simulink model "twa_parallel"  (Simulink 7.5)
settings: Solver=ode8  StartTime=0.0  StopTime=inf  FixedStep=dt  RelTol=1e-3
PreLoadFcn:
  | addpath('c:\ServoToGo');
  | addpath('d:\Projects\TwistedWireActuator\TWA_parallel_control\init_func')
InitFcn:
  | init_main_twa
  | init_scopes
  | init_twa_homing
  | init_twa_wires
undefined symbols (not defined in the file or in its folder): b_in_w, dt, enc_res, eq_homing, f_in_w, gear_rat, K_d, K_i, K_p, m_in_w, meas_macro_len, N_velocity, p_in_m, rm2w_homing, t_in_w, twa_enc_res, twa_flange_offset, twa_gamma, twa_gear_rat, use_twa, vel_filter_coeffs, velmex_pitch
libraries: xpclib x6, ServoToGo x3, simulink x2, dspswit3 x1
CloseFcn:
  | rtwprivate ssgencode ModelCloseRequest acrochordidae_v1
settings Model: Creator=Roger  LastModifiedBy=ahronoez  BufferReuse=off
settings DataIOCC: LimitDataPoints=off  SaveFormat=StructureWithTime
settings OptimizationCC: BlockReduction=off  OptimizeBlockIOStorage=off  BufferReuse=off  ExpressionFolding=off  LocalBlockOutputs=off  InitFltsAndDblsToZero=on  OptimizeModelRefInitCode=on
settings HardwareCC: ProdIntDivRoundTo=Zero  ProdEndianess=LittleEndian  ProdHWDeviceType=Generic->32-bit x86 compatible
settings RTWCC: SystemTargetFile=xpctargetert.tlc  TemplateMakefile=xpc_ert_tmf  Description=Simulink Real-Time (ERT)  GenerateReport=on  ProcessScript=xpctargetert_make_rtw_hook  IncludeHyperlinkInReport=on  GenerateTraceInfo=on  GenerateTraceReport=on  GenerateTraceReportSl=on  GenerateTraceReportSf=on  GenerateTraceReportEml=on  RTWCompilerOptimization=On
settings xpcTargetERTCC: TargetFcnLib=ansi_tfl_table_tmw.mat  TargetFunctionLibrary=ANSI_C  UtilityFuncGeneration=Auto  ERTMultiwordTypeDef=System defined  ERTCodeCoverageTool=None  ERTMultiwordLength=256  MultiwordLength=2048  GenerateFullHeader=on  GenerateSampleERTMain=off  GenerateTestInterfaces=off  IsPILTarget=off  ModelReferenceCompliant=on  ParMdlRefBuildCompliant=on  CompOptLevelCompliant=on  IncludeMdlTerminateFcn=on  GeneratePreprocessorConditionals=Use local settings  CombineOutputUpdateFcns=off  SuppressErrorStatus=off  ERTFirstTimeCompliant=off  IncludeFileDelimiter=Auto  ERTCustomFileBanners=off  SupportAbsoluteTime=on  LogVarNameModifier=rt_  MatFileLogging=on  MultiInstanceERTCode=off  SupportNonFinite=on  SupportComplex=on  PurelyIntegerCode=off  SupportContinuousTime=on  SupportNonInlinedSFcns=on  SupportVariableSizeSignals=off  EnableShiftOperators=on  ParenthesesLevel=Nominal  PortableWordSizes=off  ModelStepFunctionPrototypeControlCompliant=off  CPPClassGenCompliant=off  AutosarCompliant=off  GenerateASAP2=off  ExtModeTransport=0  ExtModeStaticAlloc=off  ExtModeStaticAllocSize=1000000  ExtModeTesting=off  InlinedParameterPlacement=Hierarchical  TargetOS=BareBoardExample  MultiInstanceErrorCode=Error  RateGroupingCode=on  RootIOFormat=Individual arguments  CoverageDialogOpen=off  ERTFilePackagingFormat=Modular  PreserveExpressionOrder=off  PreserveIfCondition=off  ConvertIfToSwitch=off  PreserveExternInFcnDecls=on  EnableUserReplacementTypes=off  MemSecPackage=--- None ---  MemSecDataConstants=Default  MemSecDataIO=Default  MemSecDataInternal=Default  MemSecDataParameters=Default  MemSecFuncInitTerm=Default  MemSecFuncExecute=Default  GRTInterface=on  GlobalDataDefinition=Auto  GlobalDataReference=Auto  ModuleNamingRule=Unspecified  ERTSrcFileBannerTemplate=ert_code_template.cgt  ERTHdrFileBannerTemplate=ert_code_template.cgt  ERTDataSrcFileTemplate=ert_code_template.cgt  ERTDataHdrFileTemplate=ert_code_template.cgt  ERTCustomFileTemplate=example_file_process.tlc  SignalDisplayLevel=10  ParamTuneLevel=10  InitialValueSource=Model  RTWCAPISignals=off  RTWCAPIParams=on  RTWCAPIStates=off  GenerateErtSFunction=off  RL32ModeModifier=Real-Time  ExtMode=on  ExtModeMexFile=ext_xpc  ExtModeIntrfLevel=Level2 - Open  ExtModeArmWhenConnect=off  RL32LogTETModifier=on  RL32LogBufSizeModifier=100000  RL32IRQSourceModifier=Timer  xPCIRQSourceBoard=None/Other  xPCIOIRQSlot=-1  xpcObjCom=off  xPCGenerateASAP2=off  xPCGenerateXML=off  RL32ObjectName=tg  xPCisDownloadable=off  xPCisDefaultEnv=on  xPCisModelTimeout=on  xPCModelTimeoutSecs=5  xpcDblBuff=off  xPCLoadParamSetFile=off

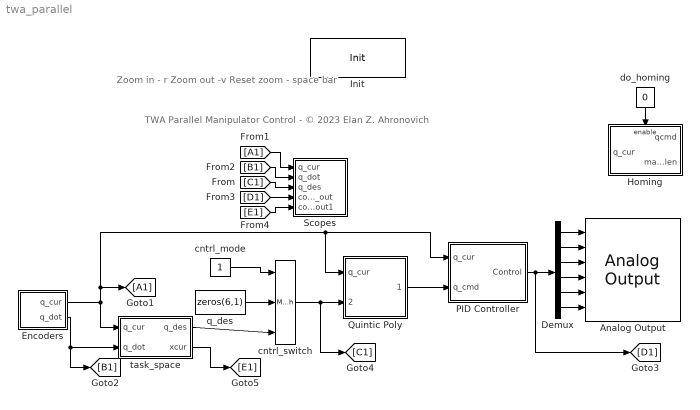
== system twa_parallel ==
  note: TWA Parallel Manipulator Control - © 2023 Elan Z. Ahronovich
  note: Zoom in - r
      | Zoom out -v
      | Reset zoom - space bar
  Analog Output : ServoToGo/Analog Output  Priority=2  channels=[0 1 2 3 4 5]
  Demux : Demux  Outputs=6
  Encoders : Subsystem
  Homing : Subsystem
  Init : ServoToGo/Init  Priority=0  sampletime=dt  baseaddress=0x300  irq_num=5  debug_flag=off  baseaddressD=0
      settings: AttributesFormatString=%<baseaddress>, IRQ: %<irq_num>\n%<sampletime>
  PID Controller : Subsystem
  Quintic Poly : Subsystem
  Scopes : Subsystem
  cntrl_mode : Constant  SampleTime=dt
  cntrl_switch : MultiPortSwitch  Inputs=2  zeroidx=off  OutDataType=fixdt(1, 16)  OutScaling=2^0  SampleTime=dt
  do_homing : Constant  Value=0  SampleTime=dt
  q_des : Constant  Value=zeros(6,1)  SampleTime=dt
  task_space : Subsystem
  wires:
  PID Controller/1(Control) -> Demux/1, [D1]
  Demux/1 -> Analog Output/1
  Demux/2 -> Analog Output/2
  Demux/3 -> Analog Output/3
  Demux/4 -> Analog Output/4
  Demux/5 -> Analog Output/5
  Demux/6 -> Analog Output/6
  Encoders/1(q_cur) -> task_space/1(q_cur), PID Controller/1(q_cur), Quintic Poly/1(q_cur), [A1]
  Encoders/2(q_dot) -> task_space/2(q_dot), [B1]
  q_des/1 -> cntrl_switch/2
  cntrl_mode/1 -> cntrl_switch/1
  Quintic Poly/1(q_cmd) -> PID Controller/2(q_cmd)
  cntrl_switch/1 -> Quintic Poly/2(q_des), [C1]
  do_homing/1 -> Homing/Enable
  task_space/1(q_des) -> cntrl_switch/3
  [C1] -> Scopes/3(q_des)
  [A1] -> Scopes/1(q_cur)
  [B1] -> Scopes/2(q_dot)
  [D1] -> Scopes/4(control_out)
  task_space/2(xcur) -> [E1]
  [E1] -> Scopes/5(control_out1)

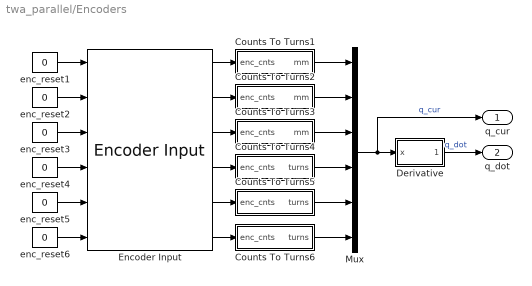
== system twa_parallel/Encoders ==
  Counts To Turns1 : Subsystem
  Counts To Turns2 : Subsystem
  Counts To Turns3 : Subsystem
  Counts To Turns4 : Subsystem
  Counts To Turns5 : Subsystem
  Counts To Turns6 : Subsystem
  Derivative : Subsystem
  Encoder Input : ServoToGo/Encoder Input  Priority=5  channels=[0 1 2 3 4 5 ]  countrev=360
  Mux : Mux  Inputs=6
  enc_reset{1..6} (6 alike) : Constant  Value=0  SampleTime=dt
  q_cur : Outport
  q_dot : Outport  Port=2
  wires:
  Encoder Input/6 -> Counts To Turns6/1(enc_cnts)
  Encoder Input/5 -> Counts To Turns5/1(enc_cnts)
  Encoder Input/4 -> Counts To Turns4/1(enc_cnts)
  Encoder Input/3 -> Counts To Turns3/1(enc_cnts)
  Encoder Input/2 -> Counts To Turns2/1(enc_cnts)
  Mux/1 -> Derivative/1(x), q_cur/1  "q_cur"
  Derivative/1(x_dot) -> q_dot/1  "q_dot"
  Encoder Input/1 -> Counts To Turns1/1(enc_cnts)
  Counts To Turns1/1(mm) -> Mux/1
  enc_reset1/1 -> Encoder Input/1
  Counts To Turns2/1(mm) -> Mux/2
  Counts To Turns3/1(mm) -> Mux/3
  Counts To Turns4/1(turns) -> Mux/4
  Counts To Turns5/1(turns) -> Mux/5
  Counts To Turns6/1(turns) -> Mux/6
  enc_reset2/1 -> Encoder Input/2
  enc_reset3/1 -> Encoder Input/3
  enc_reset4/1 -> Encoder Input/4
  enc_reset5/1 -> Encoder Input/5
  enc_reset6/1 -> Encoder Input/6

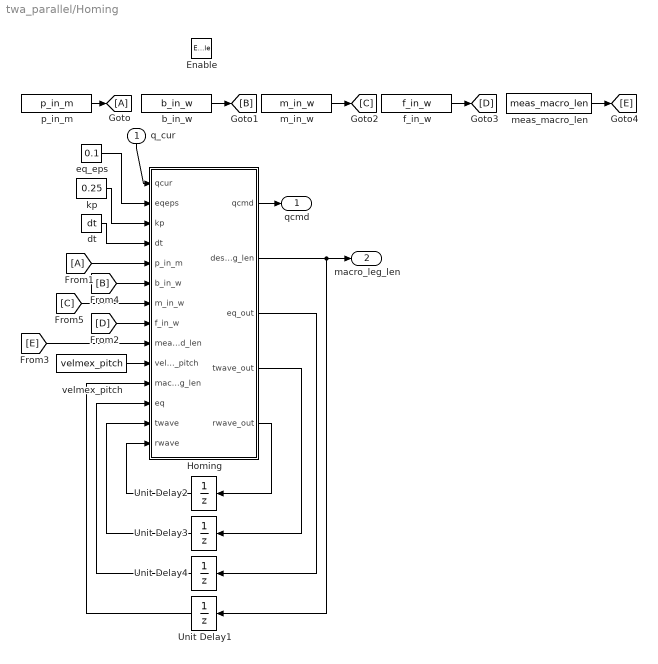
== system twa_parallel/Homing ==
  q_cur : Inport
  Enable : EnablePort
  Homing : Stateflow chart  TreatAsAtomicUnit=on
  Unit Delay1 : UnitDelay  X0=meas_macro_len  SampleTime=dt
  Unit Delay2 : UnitDelay  X0=rm2w_homing  SampleTime=dt
  Unit Delay3 : UnitDelay  X0=zeros(3,1)  SampleTime=dt
  Unit Delay4 : UnitDelay  X0=eq_homing  SampleTime=dt
  b_in_w : Constant  Value=b_in_w  SampleTime=dt
  dt : Constant  Value=dt  SampleTime=dt
  eq_eps : Constant  Value=0.1  SampleTime=dt
  f_in_w : Constant  Value=f_in_w  SampleTime=dt
  kp : Constant  Value=0.25  SampleTime=dt
  m_in_w : Constant  Value=m_in_w  SampleTime=dt
  meas_macro_len : Constant  Value=meas_macro_len  SampleTime=dt
  p_in_m : Constant  Value=p_in_m  SampleTime=dt
  velmex_pitch : Constant  Value=velmex_pitch  SampleTime=dt
  qcmd : Outport
  macro_leg_len : Outport  Port=2
  wires:
  kp/1 -> Homing/3(kp)
  dt/1 -> Homing/4(dt)
  Homing/1(qcmd) -> qcmd/1
  Homing/3(eq_out) -> Unit Delay4/1
  Homing/4(twave_out) -> Unit Delay3/1
  Unit Delay3/1 -> Homing/13(twave)
  Unit Delay4/1 -> Homing/12(eq)
  velmex_pitch/1 -> Homing/10(velmex_pitch)
  Homing/2(des_leg_len) -> Unit Delay1/1, macro_leg_len/1
  Unit Delay1/1 -> Homing/11(macro_leg_len)
  Homing/5(rwave_out) -> Unit Delay2/1
  Unit Delay2/1 -> Homing/14(rwave)
  p_in_m/1 -> [A]
  b_in_w/1 -> [B]
  [A] -> Homing/5(p_in_m)
  [B] -> Homing/6(b_in_w)
  q_cur/1 -> Homing/1(qcur)
  eq_eps/1 -> Homing/2(eqeps)
  [C] -> Homing/7(m_in_w)
  m_in_w/1 -> [C]
  f_in_w/1 -> [D]
  meas_macro_len/1 -> [E]
  [D] -> Homing/8(f_in_w)
  [E] -> Homing/9(measured_len)

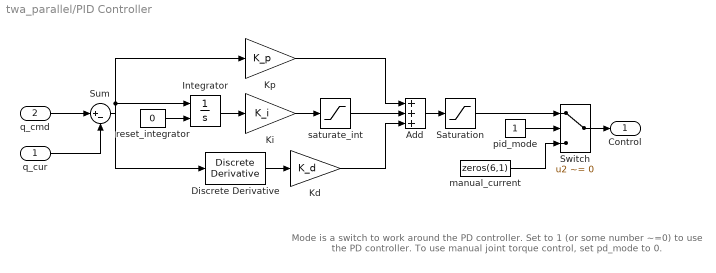
== system twa_parallel/PID Controller ==
  note: Mode is a switch to work around the PD controller.
      | Set to 1 (or some number ~=0) to use the PD
      | controller. To use manual joint torque control, set
      | pd_mode to 0.
  q_cur : Inport
  q_cmd : Inport  Port=2
  Add : Sum  Inputs=+++  SampleTime=dt
  Discrete Derivative : simulink/Discrete/Discrete Derivative  SystemSampleTime=-1  gainval=1.0  ICPrevScaledInput=0.0  OutMin=[]  OutMax=[]  OutDataType=fixdt(1, 16)  OutScaling=2^-10  DoSatur=off
  Integrator : Integrator  ExternalReset=rising
  Kd : Gain  Gain=K_d  SampleTime=dt
  Ki : Gain  Gain=K_i  SampleTime=dt
  Kp : Gain  Gain=K_p  SampleTime=dt
  Saturation : Saturate  UpperLimit=[10,10,10,2,2,2]  LowerLimit=-1*[10,10,10,2,2,2]  LinearizeAsGain=off  SampleTime=dt
  Sum : Sum  Inputs=|+-  SampleTime=dt
  Switch : Switch  Criteria=u2 ~= 0  OutDataType=fixdt(1, 16)  OutScaling=2^0  SampleTime=dt
  manual_current : Constant  Value=zeros(6,1)  SampleTime=dt
  pid_mode : Constant  SampleTime=dt
  reset_integrator : Constant  Value=0  SampleTime=dt
  saturate_int : Saturate  UpperLimit=[5,5,5,.25,0.25,0.25]  LowerLimit=-1*[5,5,5,.25,0.25,0.25]  LinearizeAsGain=off  SampleTime=dt
  Control : Outport
  wires:
  Kp/1 -> Add/1
  Kd/1 -> Add/3
  Add/1 -> Saturation/1
  q_cmd/1 -> Sum/1
  q_cur/1 -> Sum/2
  Switch/1 -> Control/1
  Saturation/1 -> Switch/1
  manual_current/1 -> Switch/3
  Ki/1 -> saturate_int/1
  saturate_int/1 -> Add/2
  Discrete Derivative/1 -> Kd/1
  Integrator/1 -> Ki/1
  Sum/1 -> Kp/1, Discrete Derivative/1, Integrator/1
  pid_mode/1 -> Switch/2
  reset_integrator/1 -> Integrator/2

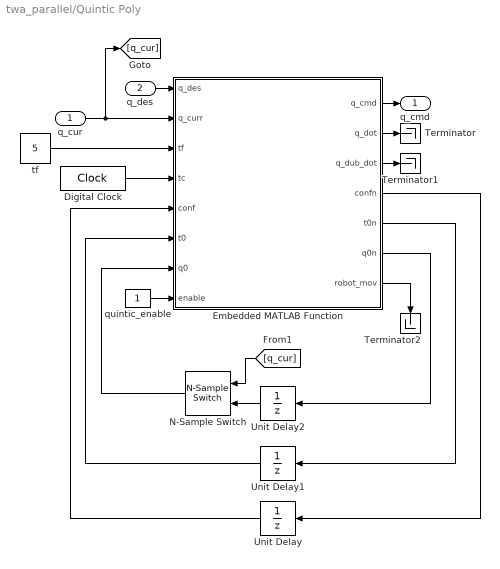
== system twa_parallel/Quintic Poly ==
  q_cur : Inport  OutDataType=fixdt(1, 16)  OutScaling=2^0
  q_des : Inport  Port=2  OutDataType=fixdt(1, 16)  OutScaling=2^0
  Digital Clock : DigitalClock  SampleTime=dt
  Embedded MATLAB Function : Stateflow chart  TreatAsAtomicUnit=on
  N-Sample Switch : dspswit3/N-Sample Switch  SystemSampleTime=-1  N=1  reset=off  TriggerType=Rising edge  Ts=dt
  Terminator : Terminator
  Terminator1 : Terminator
  Terminator2 : Terminator
  Unit Delay : UnitDelay  SampleTime=dt
  Unit Delay1 : UnitDelay  SampleTime=dt
  Unit Delay2 : UnitDelay  X0=zeros(6,1)  SampleTime=dt
  quintic_enable : Constant  SampleTime=dt
  tf : Constant  Value=5  SampleTime=dt
  q_cmd : Outport
  wires:
  Embedded MATLAB Function/4(confn) -> Unit Delay/1
  Unit Delay/1 -> Embedded MATLAB Function/5(conf)
  Embedded MATLAB Function/5(t0n) -> Unit Delay1/1
  Embedded MATLAB Function/6(q0n) -> Unit Delay2/1
  Unit Delay1/1 -> Embedded MATLAB Function/6(t0)
  Digital Clock/1 -> Embedded MATLAB Function/4(tc)
  q_des/1 -> Embedded MATLAB Function/1(q_des)
  tf/1 -> Embedded MATLAB Function/3(tf)
  quintic_enable/1 -> Embedded MATLAB Function/8(enable)
  Embedded MATLAB Function/2(q_dot) -> Terminator/1
  Embedded MATLAB Function/3(q_dub_dot) -> Terminator1/1
  N-Sample Switch/1 -> Embedded MATLAB Function/7(q0)
  Unit Delay2/1 -> N-Sample Switch/2
  [q_cur] -> N-Sample Switch/1
  Embedded MATLAB Function/7(robot_mov) -> Terminator2/1
  Embedded MATLAB Function/1(q_cmd) -> q_cmd/1
  q_cur/1 -> Embedded MATLAB Function/2(q_curr), [q_cur]

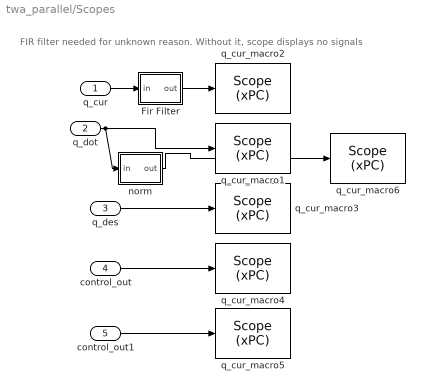
== system twa_parallel/Scopes ==
  note: FIR filter needed for unknown reason.
      |  Without it, scope displays no signals
  q_cur : Inport
  q_dot : Inport  Port=2
  q_des : Inport  Port=3
  control_out : Inport  Port=4
  control_out1 : Inport  Port=5
  Fir Filter : Subsystem
  norm : Subsystem
  q_cur_macro1 : xpclib/Misc./Scope (xPC)   SystemSampleTime=-1  scopeno=2  scopetype=Target  autostart=on  viewmode=Numerical  formatstr=qd_format  grid=on  ylimits=[0,0]  nosamples=25  noprepostsamples=0  interleave=1  triggermode=FreeRun  triggersignal=1  triggerlevel=0.0  triggerslope=Either  triggerscope=1  triggersample=0  filename=data.dat  mode=Lazy  writesize=512  autorestart=off  dynamicfilemode=off  maxwritefilesize=512*1024^2
  q_cur_macro2 : xpclib/Misc./Scope (xPC)   SystemSampleTime=-1  scopeno=1  scopetype=Target  autostart=on  viewmode=Numerical  formatstr=q_format  grid=on  ylimits=[0,0]  nosamples=25  noprepostsamples=0  interleave=1  triggermode=FreeRun  triggersignal=1  triggerlevel=0.0  triggerslope=Either  triggerscope=1  triggersample=0  filename=data.dat  mode=Lazy  writesize=512  autorestart=off  dynamicfilemode=off  maxwritefilesize=512*1024^2
  q_cur_macro3 : xpclib/Misc./Scope (xPC)   SystemSampleTime=-1  scopeno=3  scopetype=Target  autostart=on  viewmode=Numerical  formatstr=qdes_format  grid=on  ylimits=[0,0]  nosamples=25  noprepostsamples=0  interleave=1  triggermode=FreeRun  triggersignal=1  triggerlevel=0.0  triggerslope=Either  triggerscope=1  triggersample=0  filename=data.dat  mode=Lazy  writesize=512  autorestart=off  dynamicfilemode=off  maxwritefilesize=512*1024^2
  q_cur_macro4 : xpclib/Misc./Scope (xPC)   SystemSampleTime=-1  scopeno=4  scopetype=Target  autostart=on  viewmode=Numerical  formatstr=qcmd_format  grid=on  ylimits=[0,0]  nosamples=25  noprepostsamples=0  interleave=1  triggermode=FreeRun  triggersignal=1  triggerlevel=0.0  triggerslope=Either  triggerscope=1  triggersample=0  filename=data.dat  mode=Lazy  writesize=512  autorestart=off  dynamicfilemode=off  maxwritefilesize=512*1024^2
  q_cur_macro5 : xpclib/Misc./Scope (xPC)   SystemSampleTime=-1  scopeno=5  scopetype=Target  autostart=on  viewmode=Numerical  formatstr=xcur_format  grid=on  ylimits=[0,0]  nosamples=25  noprepostsamples=0  interleave=1  triggermode=FreeRun  triggersignal=1  triggerlevel=0.0  triggerslope=Either  triggerscope=1  triggersample=0  filename=data.dat  mode=Lazy  writesize=512  autorestart=off  dynamicfilemode=off  maxwritefilesize=512*1024^2
  q_cur_macro6 : xpclib/Misc./Scope (xPC)   SystemSampleTime=-1  scopeno=6  scopetype=Target  autostart=on  viewmode=Numerical  formatstr='qdot any %8i'  grid=on  ylimits=[0,0]  nosamples=25  noprepostsamples=0  interleave=1  triggermode=FreeRun  triggersignal=1  triggerlevel=0.0  triggerslope=Either  triggerscope=1  triggersample=0  filename=data.dat  mode=Lazy  writesize=512  autorestart=off  dynamicfilemode=off  maxwritefilesize=512*1024^2
  wires:
  Fir Filter/1(out) -> q_cur_macro2/1
  q_cur/1 -> Fir Filter/1(in)
  q_des/1 -> q_cur_macro3/1
  control_out/1 -> q_cur_macro4/1
  control_out1/1 -> q_cur_macro5/1
  q_dot/1 -> norm/1(in), q_cur_macro1/1
  norm/1(out) -> q_cur_macro6/1

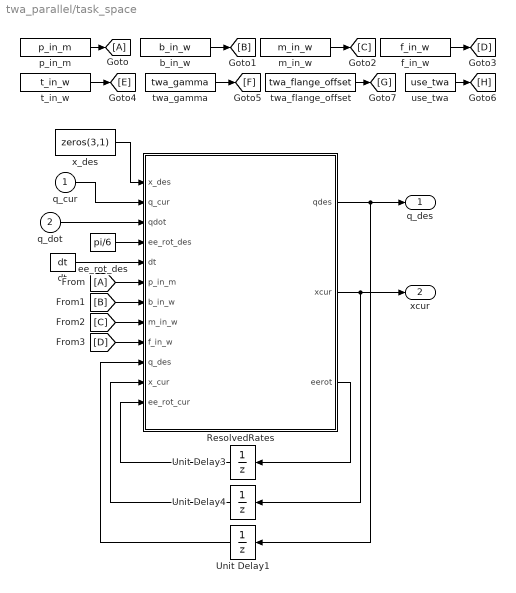
== system twa_parallel/task_space ==
  q_cur : Inport
  q_dot : Inport  Port=2
  ResolvedRates : Stateflow chart  TreatAsAtomicUnit=on
  Unit Delay1 : UnitDelay  X0=zeros(6,1)  SampleTime=dt
  Unit Delay3 : UnitDelay  X0=pi/6  SampleTime=dt
  Unit Delay4 : UnitDelay  X0=zeros(3,1)  SampleTime=dt
  b_in_w : Constant  Value=b_in_w  SampleTime=dt
  dt : Constant  Value=dt  SampleTime=dt
  ee_rot_des : Constant  Value=pi/6  SampleTime=dt
  f_in_w : Constant  Value=f_in_w  SampleTime=dt
  m_in_w : Constant  Value=m_in_w  SampleTime=dt
  p_in_m : Constant  Value=p_in_m  SampleTime=dt
  t_in_w : Constant  Value=t_in_w  SampleTime=dt
  twa_flange_offset : Constant  Value=twa_flange_offset  SampleTime=dt
  twa_gamma : Constant  Value=twa_gamma  SampleTime=dt
  use_twa : Constant  Value=use_twa  SampleTime=dt
  x_des : Constant  Value=zeros(3,1)  SampleTime=dt
  q_des : Outport
  xcur : Outport  Port=2
  wires:
  p_in_m/1 -> [A]
  b_in_w/1 -> [B]
  m_in_w/1 -> [C]
  f_in_w/1 -> [D]
  t_in_w/1 -> [E]
  twa_gamma/1 -> [F]
  twa_flange_offset/1 -> [G]
  use_twa/1 -> [H]
  ResolvedRates/3(eerot) -> Unit Delay3/1
  Unit Delay3/1 -> ResolvedRates/12(ee_rot_cur)
  ResolvedRates/2(xcur) -> Unit Delay4/1, xcur/1
  Unit Delay4/1 -> ResolvedRates/11(x_cur)
  x_des/1 -> ResolvedRates/1(x_des)
  ee_rot_des/1 -> ResolvedRates/4(ee_rot_des)
  [A] -> ResolvedRates/6(p_in_m)
  [B] -> ResolvedRates/7(b_in_w)
  [C] -> ResolvedRates/8(m_in_w)
  [D] -> ResolvedRates/9(f_in_w)
  dt/1 -> ResolvedRates/5(dt)
  ResolvedRates/1(qdes) -> Unit Delay1/1, q_des/1
  q_dot/1 -> ResolvedRates/3(qdot)
  Unit Delay1/1 -> ResolvedRates/10(q_des)
  q_cur/1 -> ResolvedRates/2(q_cur)

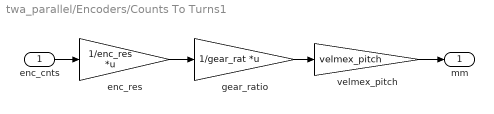
== system twa_parallel/Encoders/Counts To Turns1 ==
  enc_cnts : Inport
  enc_res : Gain  Gain=1/enc_res  Multiplication=Matrix(K*u)  SampleTime=dt
  gear_ratio : Gain  Gain=1/gear_rat  Multiplication=Matrix(K*u)  SampleTime=dt
  velmex_pitch : Gain  Gain=velmex_pitch  SampleTime=dt
  mm : Outport
  wires:
  enc_res/1 -> gear_ratio/1
  enc_cnts/1 -> enc_res/1
  gear_ratio/1 -> velmex_pitch/1
  velmex_pitch/1 -> mm/1

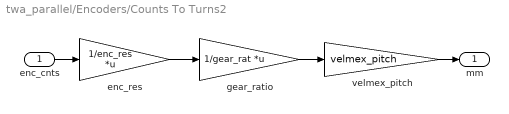
== system twa_parallel/Encoders/Counts To Turns2 ==
  enc_cnts : Inport
  enc_res : Gain  Gain=1/enc_res  Multiplication=Matrix(K*u)  SampleTime=dt
  gear_ratio : Gain  Gain=1/gear_rat  Multiplication=Matrix(K*u)  SampleTime=dt
  velmex_pitch : Gain  Gain=velmex_pitch  SampleTime=dt
  mm : Outport
  wires:
  gear_ratio/1 -> velmex_pitch/1
  enc_cnts/1 -> enc_res/1
  enc_res/1 -> gear_ratio/1
  velmex_pitch/1 -> mm/1

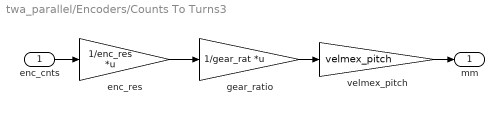
== system twa_parallel/Encoders/Counts To Turns3 ==
  enc_cnts : Inport
  enc_res : Gain  Gain=1/enc_res  Multiplication=Matrix(K*u)  SampleTime=dt
  gear_ratio : Gain  Gain=1/gear_rat  Multiplication=Matrix(K*u)  SampleTime=dt
  velmex_pitch : Gain  Gain=velmex_pitch  SampleTime=dt
  mm : Outport
  wires:
  enc_res/1 -> gear_ratio/1
  enc_cnts/1 -> enc_res/1
  gear_ratio/1 -> velmex_pitch/1
  velmex_pitch/1 -> mm/1

== system twa_parallel/Encoders/Counts To Turns4 ==
  enc_cnts : Inport
  enc_res : Gain  Gain=1/twa_enc_res  Multiplication=Matrix(K*u)  SampleTime=dt
  gear_ratio : Gain  Gain=1/twa_gear_rat  Multiplication=Matrix(K*u)  SampleTime=dt
  turns : Outport
  wires:
  gear_ratio/1 -> turns/1
  enc_cnts/1 -> enc_res/1
  enc_res/1 -> gear_ratio/1

== system twa_parallel/Encoders/Counts To Turns5 ==
  enc_cnts : Inport
  enc_res : Gain  Gain=1/twa_enc_res  Multiplication=Matrix(K*u)  SampleTime=dt
  gear_ratio : Gain  Gain=1/twa_gear_rat  Multiplication=Matrix(K*u)  SampleTime=dt
  turns : Outport
  wires:
  enc_res/1 -> gear_ratio/1
  enc_cnts/1 -> enc_res/1
  gear_ratio/1 -> turns/1

== system twa_parallel/Encoders/Counts To Turns6 ==
  enc_cnts : Inport
  enc_res : Gain  Gain=1/twa_enc_res  Multiplication=Matrix(K*u)  SampleTime=dt
  gear_ratio : Gain  Gain=1/twa_gear_rat  Multiplication=Matrix(K*u)  SampleTime=dt
  turns : Outport
  wires:
  gear_ratio/1 -> turns/1
  enc_cnts/1 -> enc_res/1
  enc_res/1 -> gear_ratio/1

== system twa_parallel/Encoders/Derivative ==
  x : Inport
  Discrete Derivative : simulink/Discrete/Discrete Derivative  SystemSampleTime=-1  gainval=1.0  ICPrevScaledInput=0.0  OutMin=[]  OutMax=[]  OutDataType=fixdt(1, 16)  OutScaling=2^-10  DoSatur=off
  Fir Filter : Subsystem
  x_dot : Outport
  wires:
  Fir Filter/1(out) -> Discrete Derivative/1
  x/1 -> Fir Filter/1(in)
  Discrete Derivative/1 -> x_dot/1

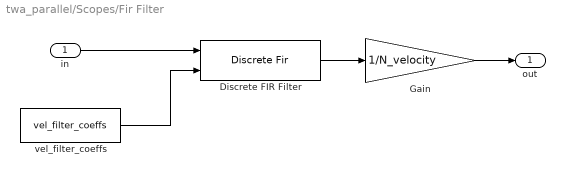
== system twa_parallel/Scopes/Fir Filter ==
  in : Inport
  Discrete FIR Filter : DiscreteFir  CoefSource=Input port  SampleTime=dt
  Gain : Gain  Gain=1/N_velocity  SampleTime=dt
  vel_filter_coeffs : Constant  Value=vel_filter_coeffs  SampleTime=dt
  out : Outport
  wires:
  in/1 -> Discrete FIR Filter/1
  Gain/1 -> out/1
  vel_filter_coeffs/1 -> Discrete FIR Filter/2
  Discrete FIR Filter/1 -> Gain/1

== system twa_parallel/Scopes/norm ==
  in : Inport
  Embedded MATLAB Function : Stateflow chart  TreatAsAtomicUnit=on
  out : Outport
  wires:
  Embedded MATLAB Function/1(y) -> out/1
  in/1 -> Embedded MATLAB Function/1(u)

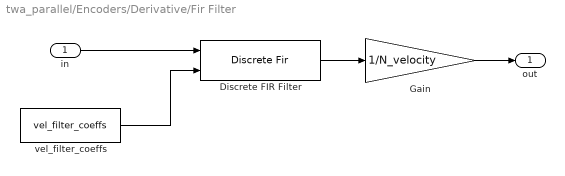
== system twa_parallel/Encoders/Derivative/Fir Filter ==
  in : Inport
  Discrete FIR Filter : DiscreteFir  CoefSource=Input port  SampleTime=dt
  Gain : Gain  Gain=1/N_velocity  SampleTime=dt
  vel_filter_coeffs : Constant  Value=vel_filter_coeffs  SampleTime=dt
  out : Outport
  wires:
  in/1 -> Discrete FIR Filter/1
  Gain/1 -> out/1
  vel_filter_coeffs/1 -> Discrete FIR Filter/2
  Discrete FIR Filter/1 -> Gain/1

== matlab function Scopes/norm/Embedded MATLAB Function ==
  data: u input double; y output double
function y = fcn(u)
%#eml

y = ~any(u);

== matlab function Homing/Homing ==
  data: qcur input double; eqeps input double; qcmd output double; des_leg_len output double; kp input double; dt input double; p_in_m input double; b_in_w input double; m_in_w input double; f_in_w input double; measured_len input double; velmex_pitch input double; macro_leg_len input double; eq input double; eq_out output double; twave_out output double; rwave_out output double; twave input double; rwave input double
function [qcmd,des_leg_len,eq_out,twave_out,rwave_out] = fcn(qcur,eqeps,kp,...
    dt,p_in_m,b_in_w,m_in_w,f_in_w,measured_len,velmex_pitch,macro_leg_len,...
    eq,twave,rwave)
%#eml
qcmd = qcur;

z0 = [0 0 1]';

% moving platform vertex locations
p_in_w = twave*ones(1,3) + rwave*p_in_m;

if norm(eq) > eqeps
    %% instantaneous direct kinematics jacobian
    % vector from base vertex to moving platform vertex
    n1hat = (p_in_w(:,1)-b_in_w(:,1))./norm(b_in_w(:,1) - p_in_w(:,1));
    n2hat = (p_in_w(:,2)-b_in_w(:,2))./norm(b_in_w(:,2) - p_in_w(:,2));
    n3hat = (p_in_w(:,3)-b_in_w(:,3))./norm(b_in_w(:,3) - p_in_w(:,3));
    
    a13 = z0'*(cross(rwave*p_in_m(:,1),n1hat));
    a23 = z0'*(cross(rwave*p_in_m(:,2),n2hat));
    a33 = z0'*(cross(rwave*p_in_m(:,3),n3hat));
    
    idk_jac = [n1hat(1,1) n1hat(2,1) a13; ...
               n2hat(1,1) n2hat(2,1) a23; ...
               n3hat(1,1) n3hat(2,1) a33];
    
    %% instantaneous inverse kinematics jacobian
    % micro actuator (TWA) lengths
    q1_mu = norm(b_in_w(:,1) - m_in_w(:,1));
    q2_mu = norm(b_in_w(:,2) - m_in_w(:,2));
    q3_mu = norm(b_in_w(:,3) - m_in_w(:,3));
    
    % vector from base vertex to twa motor attachment point
    l1_hat = (m_in_w(:,1) - b_in_w(:,1)) ./ norm(m_in_w(:,1) - b_in_w(:,1));
    l2_hat = (m_in_w(:,2) - b_in_w(:,2)) ./ norm(m_in_w(:,2) - b_in_w(:,2));
    l3_hat = (m_in_w(:,3) - b_in_w(:,3)) ./ norm(m_in_w(:,3) - b_in_w(:,3));
    
    % distance from micro actuator attachmnet point (m_i) to flexure rotation
    %center (f_i)
    a1 = norm(m_in_w(:,1) - f_in_w(:,1));
    a2 = norm(m_in_w(:,2) - f_in_w(:,2));
    a3 = norm(m_in_w(:,3) - f_in_w(:,3));
    
    % distance from flexure rotation center (f_i) to base vertex
    c1 = norm(b_in_w(:,1)-f_in_w(:,1));
    c2 = norm(b_in_w(:,2)-f_in_w(:,2));
    c3 = norm(b_in_w(:,3)-f_in_w(:,3));
    
    % term to paramterize angle between a_i and qimu, delta
    h1 = (c1^2 - a1^2 - q1_mu^2)/(-2*a1*q1_mu);
    h2 = (c2^2 - a2^2 - q2_mu^2)/(-2*a2*q2_mu);
    h3 = (c3^2 - a3^2 - q3_mu^2)/(-2*a3*q3_mu);
    
    % time derivatives
    h1dot = (4*a1*q1_mu^2 + (c1^2 - a1^2 - q1_mu^2)*2*a1) / (4*a1^2*q1_mu^2);
    h2dot = (4*a2*q2_mu^2 + (c2^2 - a2^2 - q2_mu^2)*2*a2) / (4*a2^2*q2_mu^2);
    h3dot = (4*a3*q3_mu^2 + (c3^2 - a3^2 - q3_mu^2)*2*a3) / (4*a3^2*q3_mu^2);
    
    e1 = n1hat' * l1_hat + q1_mu*h1dot/sqrt(1-h1^2) * n1hat' * cross(z0,l1_hat);
    e2 = n2hat' * l2_hat + q2_mu*h2dot/sqrt(1-h2^2) * n2hat' * cross(z0,l2_hat);
    e3 = n3hat' * l3_hat + q3_mu*h3dot/sqrt(1-h3^2) * n3hat' * cross(z0,l3_hat);
    
    % micro motion instantaneous inverse kinematics jacobian
    b_mu = [e1 0 0;...
            0 e2 0;...
            0 0 e3];
    
    % macro motion instantaneous inverse kinematics jacobian
    b_m = eye(3);

    % combined macro-micro motion IIK jacobian
    iik_jac = [b_m,b_mu];
    
    % the full manipulator jacobian with redundancy resolution weighting
    w_mat = diag([1,1,1,1e10,1e10,1e10]);
    full_jac = (w_mat\iik_jac') / (iik_jac/w_mat*iik_jac') * idk_jac;

    %%
    % joint velocities and ee velocity proportional to joint error
    qdot = kp * eq;
    tdot = full_jac*qdot;
    
    % separate translational and rotational components of twist
    v = tdot(1:2,1);
    w = tdot(3,1);
    
    % new end effector position
    twave(1:2,1) = twave(1:2,1) + v*dt;
    
    % change in end effector orientation
    del_r = [cos(w*dt) -sin(w*dt) 0;sin(w*dt) cos(w*dt) 0;0 0 1];
    
    % new end effector orientation
    rwave = del_r*rwave;
    
    des_leg_len = zeros(3,1);
    for i = 1:3
        p_in_w(:,i) = twave + rwave*p_in_m(:,i);
        des_leg_len(i,1) = norm(p_in_w(:,i) - b_in_w(:,i));
    end
    
    eq_out = macro_leg_len - des_leg_len;
    
    % the amount each velmex slides need to move is the difference between
    % the last leg length and the new leg length
    %     qcmd(1:3,1) = (measured_len - des_leg_len)/velmex_pitch
    qcmd(1:3,1) = (des_leg_len - measured_len)/velmex_pitch;
    
    twave_out = twave;
    rwave_out = rwave;
else
    des_leg_len = macro_leg_len;
    eq_out = eq;
    twave_out = twave;
    rwave_out = rwave;
end

== matlab function task_space/ResolvedRates ==
  data: x_des input double; q_cur input double; qdot input double; ee_rot_des input double; dt input double; p_in_m input double; b_in_w input double; m_in_w input double; f_in_w input double; q_des input double; x_cur input double; ee_rot_cur input double; qdes output double; xcur output double; eerot output double
function [qdes,xcur,eerot] = redResRate(x_des,q_cur,qdot,ee_rot_des,dt,p_in_m,...
    b_in_w,m_in_w,f_in_w,q_des,x_cur,ee_rot_cur)

qdes = q_des;
xcur = x_cur;
eerot = ee_rot_cur;

% axis for jacobian definitions
z0 = [0 0 1]';

% positional error
p_del = norm(x_des - x_cur);

% desired orientation angle rotation matrix and error roation matrix
r_des = [cos(ee_rot_des) -sin(ee_rot_des) 0;sin(ee_rot_des) cos(ee_rot_des) 0;0 0 1];
r_cur = [cos(ee_rot_cur) -sin(ee_rot_cur) 0;sin(ee_rot_cur) cos(ee_rot_cur) 0;0 0 1];
r_del = r_des * r_cur';

% orientational error angle and axis
theta_e = acos((trace(r_del)-1)/2);

% error thresholds
p_epsilon = 0.01;
w_epsilon = 0.001;

% only look when all of the actuators are not moving
if ~any(qdot)
    if theta_e > w_epsilon || p_del > p_epsilon
        % moving platform vertex locations
        p_in_w = x_cur*ones(1,3) + r_cur*p_in_m;
        
        %% instantaneous direct kinematics jacobian
        % vector from base vertex to moving platform vertex
        n1hat = (p_in_w(:,1)-b_in_w(:,1))./norm(b_in_w(:,1) - p_in_w(:,1));
        n2hat = (p_in_w(:,2)-b_in_w(:,2))./norm(b_in_w(:,2) - p_in_w(:,2));
        n3hat = (p_in_w(:,3)-b_in_w(:,3))./norm(b_in_w(:,3) - p_in_w(:,3));
        
        a13 = z0'*(cross(r_cur*p_in_m(:,1),n1hat));
        a23 = z0'*(cross(r_cur*p_in_m(:,2),n2hat));
        a33 = z0'*(cross(r_cur*p_in_m(:,3),n3hat));
        
        idk_jac = [n1hat(1,1) n1hat(2,1) a13; ...
            n2hat(1,1) n2hat(2,1) a23; ...
            n3hat(1,1) n3hat(2,1) a33];
        
        %% instantaneous inverse kinematics jacobian
        % micro actuator (TWA) lengths
        q1_mu = norm(b_in_w(:,1) - m_in_w(:,1));
        q2_mu = norm(b_in_w(:,2) - m_in_w(:,2));
        q3_mu = norm(b_in_w(:,3) - m_in_w(:,3));
        
        % vector from base vertex to twa motor attachment point
        l1_hat = (m_in_w(:,1) - b_in_w(:,1)) ./ norm(m_in_w(:,1) - b_in_w(:,1));
        l2_hat = (m_in_w(:,2) - b_in_w(:,2)) ./ norm(m_in_w(:,2) - b_in_w(:,2));
        l3_hat = (m_in_w(:,3) - b_in_w(:,3)) ./ norm(m_in_w(:,3) - b_in_w(:,3));
        
        % distance from micro actuator attachmnet point (m_i) to flexure rotation
        %center (f_i)
        a1 = norm(m_in_w(:,1) - f_in_w(:,1));
        a2 = norm(m_in_w(:,2) - f_in_w(:,2));
        a3 = norm(m_in_w(:,3) - f_in_w(:,3));
        
        % distance from flexure rotation center (f_i) to base vertex
        c1 = norm(b_in_w(:,1)-f_in_w(:,1));
        c2 = norm(b_in_w(:,2)-f_in_w(:,2));
        c3 = norm(b_in_w(:,3)-f_in_w(:,3));
        
        % term to paramterize angle between a_i and qimu, delta
        h1 = (c1^2 - a1^2 - q1_mu^2)/(-2*a1*q1_mu);
        h2 = (c2^2 - a2^2 - q2_mu^2)/(-2*a2*q2_mu);
        h3 = (c3^2 - a3^2 - q3_mu^2)/(-2*a3*q3_mu);
        
        % time derivatives
        h1dot = (4*a1*q1_mu^2 + (c1^2 - a1^2 - q1_mu^2)*2*a1) / (4*a1^2*q1_mu^2);
        h2dot = (4*a2*q2_mu^2 + (c2^2 - a2^2 - q2_mu^2)*2*a2) / (4*a2^2*q2_mu^2);
        h3dot = (4*a3*q3_mu^2 + (c3^2 - a3^2 - q3_mu^2)*2*a3) / (4*a3^2*q3_mu^2);
        
        e1 = n1hat' * l1_hat + q1_mu*h1dot/sqrt(1-h1^2) * n1hat' * cross(z0,l1_hat);
        e2 = n2hat' * l2_hat + q2_mu*h2dot/sqrt(1-h2^2) * n2hat' * cross(z0,l2_hat);
        e3 = n3hat' * l3_hat + q3_mu*h3dot/sqrt(1-h3^2) * n3hat' * cross(z0,l3_hat);
        
        % micro motion instantaneous inverse kinematics jacobian
        b_mu = [e1 0 0;...
            0 e2 0;...
            0 0 e3];
        
        % macro motion instantaneous inverse kinematics jacobian
        b_m = eye(3);
        
        % combined macro-micro motion IIK jacobian
        iik_jac = [b_m,b_mu];
        
        % the full manipulator jacobian with redundancy resolution weighting
        w_mat = diag([1,1,1,1e10,1e10,1e10]);
        full_jac = (w_mat\iik_jac') / (iik_jac/w_mat*iik_jac') * idk_jac;
        
        % positional error direction
        p_ep_hat = (x_des-x_cur)/p_del;
        
        % orientational error axis
        if theta_e ~= 0
            me = (1/(2*sin(theta_e)))*[r_del(3,2)-r_del(2,3);...
                r_del(1,3)-r_del(3,1);...
                r_del(2,1)-r_del(1,2)];
        else
            me = z0;
        end
        
        % inverse kinematics based on pose error
        vmax = 1; %[mm/s]
        vmin = 0.02;
        wmin = 0.001;
        wmax = 0.05;
        p_lambda = 3;
        w_lambda = 3;
        vdot = 0;
        wdot = 0;
        
        if p_del ~=0
            if p_del/p_epsilon <= p_lambda
                vdot = vmin + (((vmax-vmin)*(p_del-p_epsilon))/(p_epsilon*(p_lambda-1)));
            else
                vdot = vmax;
            end
        end
        
        if theta_e ~= 0
            if theta_e/w_epsilon <= w_lambda && theta_e ~= 0
                wdot = wmin + (((wmax-wmin)*(theta_e-w_epsilon))/(w_epsilon*(w_lambda-1)));
            else
                wdot = wmax;
            end
        end
        
        v = vdot * p_ep_hat;
        w = wdot * me;
        
        qdot = full_jac * [v(1:2);w(3)];
        deltaq = qdot * dt;
        qdes = q_cur + deltaq;
       
        xcur = x_cur + v * dt;
        eerot = ee_rot_cur + w(3) * dt;
    else
        qdes = q_cur;
        xcur = x_cur;
        % check this for angle or rotation matrix
        eerot = ee_rot_cur;
    end
end

end

== matlab function Quintic Poly/Embedded MATLAB Function ==
  data: q_cmd output double; q_des input double; q_curr input double; tf input double; tc input double; q_dot output double; q_dub_dot output double; conf input double; confn output double; t0 input double; t0n output double; q0n output double; q0 input double; enable input double; robot_mov output double
function [q_cmd,q_dot,q_dub_dot,confn,t0n,q0n,robot_mov] = fifth_order_p(q_des,q_curr,tf,tc,conf,t0,q0,enable)
% number of actuators
n = size(q_des,1);

robot_mov = 0;
eta = q_des - q0;

if enable
    if (eta)'*(eta) > 0
        % conf = 0 means that the 5th order poly
        % is not configured for the desired trajectory.
        % Therefore, the block is initialized.
        if conf == 0               
            q0n = q0;               
            t0n = tc;               
            confn = 1;
            q_cmd = q0;
            q_dot = zeros(n,1);
            q_dub_dot = zeros(n,1);
        else
            q0n = q0;
            t0n = t0;
            confn = conf;
            
            % 5th order polynomial
            a0 = q0;
            a4 = -15*(eta);
            a3 = -2/3 * a4;
            a5 = -2/5 * a4;
            t = tc-t0;
            tau = t/tf;
            
            if t < tf
                robot_mov = 1;
                q_cmd = a0 + a3 * tau^3 + a4 * tau^4 + a5 * tau^5;
                q_dot = 3*a3*t^2/tf^3 + 4*a4*t^3/tf^4 + 5*a5*t^4/tf^5;
                q_dub_dot = 6*a3*t/tf^3 + 12*a4*t^2/tf^4 + 20*a5*t^3/tf^5;
            else
                q_cmd = q_des;
                q_dot = zeros(n,1);
                q_dub_dot = zeros(n,1);
                q0n = q_des;
            end
        end
    else
        q_cmd = q_des;
        q_dot = zeros(n,1);
        q_dub_dot = zeros(n,1);
        confn = 0;
        q0n = q0;
        t0n = t0;
    end
else
    % Configuration space is not used (pdot = 0).
    q_cmd = q_des;
    q_dot = zeros(n,1);
    q_dub_dot = zeros(n,1);       % However we do want to record the current
    confn = 0;                  % position in order to be ready as soon
    t0n = tc;                   % as the enable becomes 1.
    q0n = q_curr;
end
%------------------------------------------------------------------------
